simulink model "QPSK_Tx_HDL"  (R2017b)
settings: Solver=FixedStepDiscrete  StartTime=0.0  StopTime=inf  RelTol=1e-3
PreLoadFcn:
  | sdrzQPSKTxFPGA_params = QPSK_Tx_HDL_init;
InitFcn:
  | sdrzQPSKTxFPGA_params = QPSK_Tx_HDL_init;
libraries: hdlsllib x3, dspsigops x2, adirfsom_lib x1, commrandsrc3 x1, commsequence2 x1, dspmlti4 x1, commdigbbndpm3 x1
CloseFcn:
  | clear sdrzQPSKTxFPGA_params;
Description:
  | This model is used to generate a targeted .bit for an SDR platform
settings Model: DataTypeOverride=Off  ModifiedByFormat=The MathWorks Inc.  SimulationMode=accelerator  Creator=The MathWorks, Inc.  LastModifiedBy=The MathWorks Inc.
settings DataIOCC: LimitDataPoints=on  SaveFormat=Array  SaveOutput=off  SaveTime=off
settings OptimizationCC: BlockReduction=off  ConditionallyExecuteInputs=off  DefaultParameterBehavior=Inlined  LifeSpan=inf
settings DebuggingCC: AlgebraicLoopMsg=error  UnderspecifiedInitializationDetection=Classic  MergeDetectMultiDrivingBlocksExec=none  SolverPrmCheckMsg=warning  MultiTaskDSMMsg=warning  MultiTaskCondExecSysMsg=none  SingleTaskRateTransMsg=error  ParameterPrecisionLossMsg=none  AllowSymbolicDim=off  StateNameClashWarn=warning  SFUnexpectedBacktrackingDiag=warning  SFNoUnconditionalDefaultTransitionDiag=warning  SFExecutionAtInitializationDiag=none
settings HardwareCC: ProdBitPerPointer=32  ProdBitPerSizeT=32  ProdBitPerPtrDiffT=32  ProdLargestAtomicFloat=None  ProdIntDivRoundTo=Undefined  ProdEndianess=Unspecified  ProdWordSize=32  ProdHWDeviceType=ASIC/FPGA->ASIC/FPGA  TargetBitPerPointer=64  TargetBitPerSizeT=64  TargetBitPerPtrDiffT=64  TargetLongLongMode=on  TargetIntDivRoundTo=Zero  TargetEndianess=LittleEndian  TargetWordSize=64  TargetHWDeviceType=Generic->MATLAB Host Computer  ProdEqTarget=off
settings ModelReferenceCC: PropagateSignalLabelsOutOfModel=off
settings CodeAppCC: StateflowObjectComments=on
settings GRTTargetCC: TargetLangStandard=C89/C90 (ANSI)  GeneratePreprocessorConditionals=Disable all
settings ConfigComp: CovMetricSettings=dw  CovHtmlReporting=on  CovSaveCumulativeToWorkspaceVar=on  CovSaveSingleToWorkspaceVar=on  CovExternalEMLEnable=off  CovSFcnEnable=off

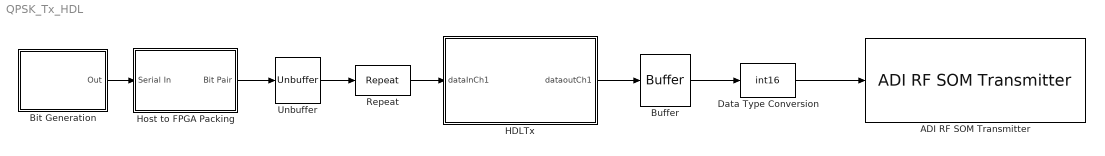
== system QPSK_Tx_HDL ==
  ADI RF SOM Transmitter : adirfsom_lib/ADI RF SOM Transmitter  IPAddress=192.168.3.2  CenterFrequencySource=Dialog  CenterFrequency=2400000000  GainSource=Dialog  Gain=-10  ChannelMapping=1  BasebandSampleRate=sdrzQPSKTxFPGA_params.RadioFrontEndSampleRate  EnableBurstMode=off  NumFramesInBurst=20  DMATimeoutValue=1  EnableTxPrimingMode=on  blockMode=Normal  LostSamplesOutputPort=off  OverflowOutputPort=off  SimulateUsing=Code generation  DataSourceSelect=Host  DDSFrequency=[ 1000000, 1000000; 1000000, 1000000 ]  DDSPhase=[ 0, 0; 0, 0 ]  DDSScale=[ 250000, 250000; 250000, 250000 ]  BypassUserLogic=on  ShowAdvancedProperties=on  ShowInternalProperties=off  subDeviceList=zynqTransmitter  sdrExecutionMode=HW  dataUDPPort=-1  ctrlUDPPort=-1  FIRCoefficientSize=[ 128; 128 ]  FIRCoefficients=[ 55, -54, 42, -126, -123, -317, -399, -581, -646, -711, -634, -507, -263, -10, 255, 424, 492, 401, 201, -84, -352, -540, -566, -423, -126, 234, 562, 738, 701, 429, -5, -490, -866, -1007, -834, -372, 266, 891, 1301, 1334, 936, 178, -733, -1524, -1917, -1731, -944, 274, 1590, 2585, 2881, 2255, 741, -1344, -3435, -4850, -4942, -3285, 197, 5169, 10923, 16509, 20932, 23375, 23375, 20932, 16509, 10923, 5169, 197, -3285, -4942, -4850, -3435, -1344, 741, 2255, 2881, 2585, 1590, 274, -944, -1731, -1917, -1524, -733, 178, 936, 1334, 1301, 891, 266, -372, -834, -1007, -866, -490, -5, 429, 701, 738, 562, 234, -126, -423, -566, -540, -352, -84, 201, 401, 492, 424, 255, -10, -263, -507, -634, -711, -646, -581, -399, -317, -123, -126, 42, -54, 55; 190, -88, 329, -40, 239, -99, -24, -349, -377, -611, -573, -604, -395, -229, 66, 239, 394, 350, 227, -46, -300, -534, -593, -506, -221, 137, 512, 737, 765, 526, 103, -420, -852, -1069, -947, -512, 156, 841, 1341, 1450, 1100, 333, -638, -1531, -2028, -1922, -1152, 115, 1544, 2677, 3099, 2535, 997, -1205, -3479, -5095, -5345, -3750, -199, 4965, 11002, 16895, 21580, 24172, 24172, 21580, 16895, 11002, 4965, -199, -3750, -5345, -5095, -3479, -1205, 997, 2535, 3099, 2677, 1544, 115, -1152, -1922, -2028, -1531, -638, 333, 1100, 1450, 1341, 841, 156, -512, -947, -1069, -852, -420, 103, 526, 765, 737, 512, 137, -221, -506, -593, -534, -300, -46, 227, 350, 394, 239, 66, -229, -395, -604, -573, -611, -377, -349, -24, -99, 239, -40, 329, -88, 190 ]  FIRGain=[ 0; -12 ]  FIRDecimInterpFactor=[ 4; 4 ]  AnalogFilterCutoff=[ 3152524; 3161715 ]  FilterPathRates=[ 983040000, 122880000, 61440000, 30720000, 15360000, 3840000; 983040000, 122880000, 61440000, 30720000, 15360000, 3840000 ]  FilterDesignTypeForTx=DefaultFilter  FilterDesignTypeForRx=DefaultFilterFromOther
      settings: SourceProductName=Communications System Toolbox Support Package for Xilinx Zynq-Based Radio
  Bit Generation : Subsystem
      mask Display: disp('Bits Generation')
  Buffer : Buffer  N=4000  OutputFrames=off
  Data Type Conversion : DataTypeConversion  OutDataTypeStr=int16  ConvertRealWorld=Stored Integer (SI)
  HDLTx : Subsystem
  Host to FPGA Packing : Subsystem
  Repeat : dspsigops/Repeat  N=sdrzQPSKTxFPGA_params.Upsampling  RateOptions=Allow multirate processing  ic=0  mode=Unused parameter value
      settings: SourceProductName=DSP System Toolbox
  Unbuffer : Unbuffer
  wires:
  Unbuffer/1 -> Repeat/1
  Bit Generation/1(Out) -> Host to FPGA Packing/1(Serial In)
  Buffer/1 -> Data Type Conversion/1
  HDLTx/1(dataoutCh1) -> Buffer/1
  Host to FPGA Packing/1(Bit Pair) -> Unbuffer/1
  Repeat/1 -> HDLTx/1(dataInCh1)
  Data Type Conversion/1 -> ADI RF SOM Transmitter/1

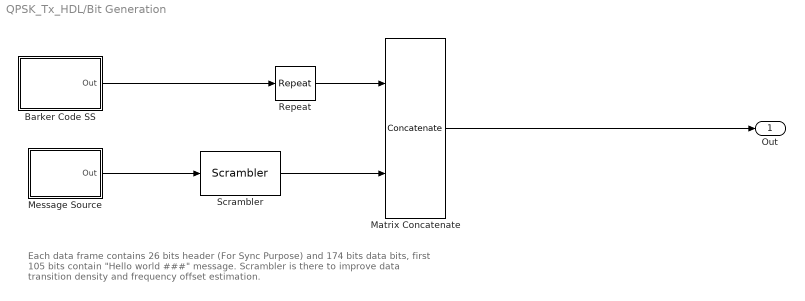
== system QPSK_Tx_HDL/Bit Generation ==
  note: Each data frame contains 26 bits header (For Sync Purpose) and 174 bits data bits,
      | first 105 bits contain "Hello world ###" message. Scrambler is there to improve data
      | transition density and frequency offset estimation.
  Barker Code SS : Subsystem
      mask Display: disp('Unipolar\nBarker Code')
  Matrix Concatenate : Concatenate  Mode=Multidimensional array
  Message Source : Subsystem
      mask Display: disp('Message\nSource')
  Repeat : dspsigops/Repeat  N=2  InputProcessing=Columns as channels (frame based)  RateOptions=Enforce single-rate processing  ic=0  mode=Unused parameter value
      settings: SourceProductName=DSP System Toolbox
  Scrambler : commsequence2/Scrambler  M=2  poly=[1 1 1 0 1]  iniStaSource=Dialog Parameter  ini_sta=[0 0 0 0]  resetViaPort=off
      settings: SourceProductName=Communications System Toolbox  SourceProductBaseCode=CM
  Out : Outport
  wires:
  Message Source/1(Out) -> Scrambler/1
  Scrambler/1 -> Matrix Concatenate/2
  Repeat/1 -> Matrix Concatenate/1
  Barker Code SS/1(Out) -> Repeat/1
  Matrix Concatenate/1 -> Out/1

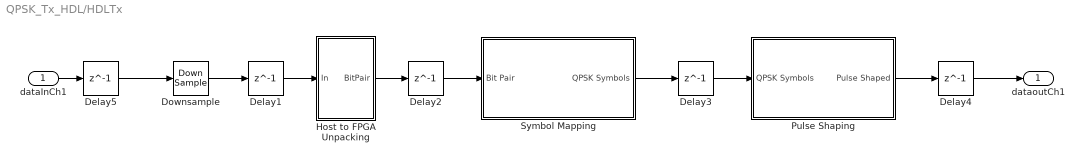
== system QPSK_Tx_HDL/HDLTx ==
  dataInCh1 : Inport
  Delay{1..5} (5 alike) : Delay  DelayLength=1  InitialCondition=0
  Downsample : DownSample  N=sdrzQPSKTxFPGA_params.Upsampling  RateOptions=Allow multirate processing
  Host to FPGA Unpacking : Subsystem
  Pulse Shaping : Subsystem
  Symbol Mapping : Subsystem
  dataoutCh1 : Outport
  wires:
  Delay3/1 -> Pulse Shaping/1(QPSK Symbols)
  Pulse Shaping/1(Pulse Shaped) -> Delay4/1
  Delay4/1 -> dataoutCh1/1
  Delay1/1 -> Host to FPGA Unpacking/1(In)
  dataInCh1/1 -> Delay5/1
  Delay2/1 -> Symbol Mapping/1(Bit Pair)
  Host to FPGA Unpacking/1(BitPair) -> Delay2/1
  Symbol Mapping/1(QPSK Symbols) -> Delay3/1
  Delay5/1 -> Downsample/1
  Downsample/1 -> Delay1/1

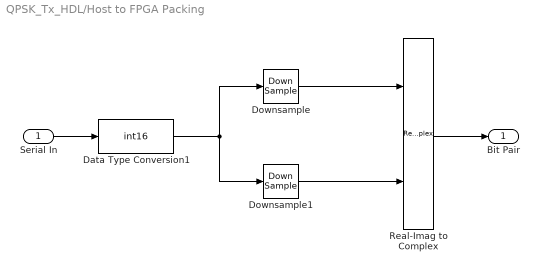
== system QPSK_Tx_HDL/Host to FPGA Packing ==
  Serial In : Inport
  Data Type Conversion1 : DataTypeConversion  OutDataTypeStr=int16
  Downsample : DownSample  RateOptions=Allow multirate processing
  Downsample1 : DownSample  phase=1  RateOptions=Allow multirate processing
  Real-Imag to Complex : RealImagToComplex
  Bit Pair : Outport
  wires:
  Downsample/1 -> Real-Imag to Complex/1
  Serial In/1 -> Data Type Conversion1/1
  Data Type Conversion1/1 -> Downsample1/1, Downsample/1
  Downsample1/1 -> Real-Imag to Complex/2
  Real-Imag to Complex/1 -> Bit Pair/1

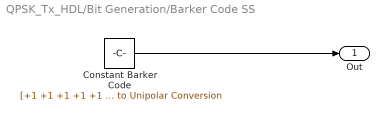
== system QPSK_Tx_HDL/Bit Generation/Barker Code SS ==
  Constant Barker Code : Constant  Value=|  VectorParams1D=off  OutDataTypeStr=double
      | [+1 +1 +1 +1 +1 -1 -1 +1 +1 -1 +1 -1 +1
      | ].' > 0  % Bipolar to Unipolar Conversion
  Out : Outport
  wires:
  Constant Barker Code/1 -> Out/1

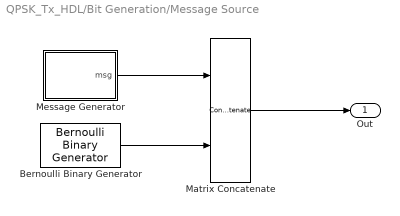
== system QPSK_Tx_HDL/Bit Generation/Message Source ==
  Bernoulli Binary Generator : commrandsrc3/Bernoulli Binary Generator  ProbabilityOfZero=0.5  SeedSource=Parameter  Seed=61  SampleTime=sdrzQPSKTxFPGA_params.FrameTime / (sdrzQPSKTxFPGA_params.DataLength - sdrzQPSKTxFPGA_params.MsgLength)  SamplesPerFrame=sdrzQPSKTxFPGA_params.DataLength - sdrzQPSKTxFPGA_params.MsgLength  OutputDataType=double  SimulateUsing=Interpreted execution
  Matrix Concatenate : Concatenate  Mode=Multidimensional array
  Message Generator : MATLAB Function  TreatAsAtomicUnit=on
  Out : Outport
  wires:
  Matrix Concatenate/1 -> Out/1
  Bernoulli Binary Generator/1 -> Matrix Concatenate/2
  Message Generator/1(msg) -> Matrix Concatenate/1

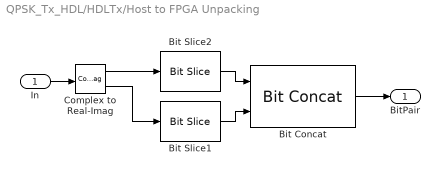
== system QPSK_Tx_HDL/HDLTx/Host to FPGA Unpacking ==
  In : Inport
  Bit Concat : hdlsllib/Logic and Bit Operations/Bit Concat  numInputs=2
      settings: SourceProductName=HDL Coder  SourceProductBaseCode=HD
  Bit Slice1 : hdlsllib/Logic and Bit Operations/Bit Slice  lidx=0  ridx=0
  Bit Slice2 : hdlsllib/Logic and Bit Operations/Bit Slice  lidx=0  ridx=0
  Complex to Real-Imag : ComplexToRealImag
  BitPair : Outport
  wires:
  Complex to Real-Imag/1 -> Bit Slice2/1
  In/1 -> Complex to Real-Imag/1
  Complex to Real-Imag/2 -> Bit Slice1/1
  Bit Slice2/1 -> Bit Concat/1
  Bit Slice1/1 -> Bit Concat/2
  Bit Concat/1 -> BitPair/1

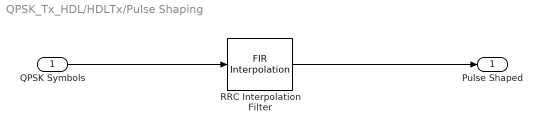
== system QPSK_Tx_HDL/HDLTx/Pulse Shaping ==
  QPSK Symbols : Inport
  RRC Interpolation Filter : dspmlti4/FIR Interpolation  FilterSource=Dialog parameters  h=sdrzQPSKTxFPGA_params.TransmitterFilterCoefficients  L=sdrzQPSKTxFPGA_params.Upsampling  FilterObject=Htxrc  framing=Allow multirate processing  outputBufInitCond=0  roundingMode=Floor  overflowMode=off  firstCoeffMode=Specify word length  firstCoeffWordLength=16  firstCoeffFracLength=15  firstCoeffDataTypeStr=fixdt(1,16)  firstCoeffMin=[]  firstCoeffMax=[]  firstCoeffLastDataTypeStr=fixdt(1,16)  prodOutputMode=Binary point scaling  prodOutputWordLength=31  prodOutputFracLength=29  prodOutputDataTypeStr=fixdt(1,31,29)  prodOutputLastDataTypeStr=fixdt(1,31,29)  accumMode=Binary point scaling  accumWordLength=33  accumFracLength=29  accumDataTypeStr=fixdt(1,33,29)  accumLastDataTypeStr=fixdt(1,33,29)  outputMode=Binary point scaling  outputWordLength=16  outputFracLength=14  outputDataTypeStr=fixdt(1,16,14)  outputMin=[]  outputMax=[]  outputLastDataTypeStr=fixdt(1,16,14)
      settings: SourceProductName=DSP System Toolbox
  Pulse Shaped : Outport
  wires:
  QPSK Symbols/1 -> RRC Interpolation Filter/1
  RRC Interpolation Filter/1 -> Pulse Shaped/1

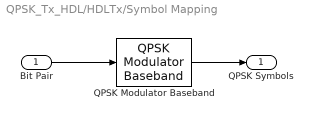
== system QPSK_Tx_HDL/HDLTx/Symbol Mapping ==
  Bit Pair : Inport
  QPSK Modulator Baseband : commdigbbndpm3/QPSK Modulator Baseband  InType=Integer  Enc=Gray  Ph=pi/4  outDtype=Fixed-point  outWordLen=16  outUDDataType=sfix(16)  outFracLenMode=User-defined  outFracLen=15  outDataTypeStr=fixdt(1,16,15)  outLastDataTypeStr=fixdt(1,16,15)
  QPSK Symbols : Outport
  wires:
  QPSK Modulator Baseband/1 -> QPSK Symbols/1
  Bit Pair/1 -> QPSK Modulator Baseband/1

== matlab function QPSK_Tx_HDL/Bit Generation/Message Source/Message Generator ==
  data: msg output size=[sdrzQPSKTxFPGA_params.MsgLength,1]
function msg = genMsg
%#codegen
persistent msgStrSet count;
if isempty(msgStrSet)
    count = 0;
    msgStrSet = ['Hello world 000';...
              'Hello world 001';...
              'Hello world 002';...
              'Hello world 003';...
              'Hello world 004';...
              'Hello world 005';...
              'Hello world 006';...
              'Hello world 007';...
              'Hello world 008';...
              'Hello world 009';...
              'Hello world 010';...
              'Hello world 011';...
              'Hello world 012';...
              'Hello world 013';...
              'Hello world 014';...
              'Hello world 015';...
              'Hello world 016';...
              'Hello world 017';...
              'Hello world 018';...
              'Hello world 019';...
              'Hello world 020';...
              'Hello world 021';...
              'Hello world 022';...
              'Hello world 023';...
              'Hello world 024';...
              'Hello world 025';...
              'Hello world 026';...
              'Hello world 027';...
              'Hello world 028';...
              'Hello world 029';...
              'Hello world 030';...
              'Hello world 031';...
              'Hello world 032';...
              'Hello world 033';...
              'Hello world 034';...
              'Hello world 035';...
              'Hello world 036';...
              'Hello world 037';...
              'Hello world 038';...
              'Hello world 039';...
              'Hello world 040';...
              'Hello world 041';...
              'Hello world 042';...
              'Hello world 043';...
              'Hello world 044';...
              'Hello world 045';...
              'Hello world 046';...
              'Hello world 047';...
              'Hello world 048';...
              'Hello world 049';...
              'Hello world 050';...
              'Hello world 051';...
              'Hello world 052';...
              'Hello world 053';...
              'Hello world 054';...
              'Hello world 055';...
              'Hello world 056';...
              'Hello world 057';...
              'Hello world 058';...
              'Hello world 059';...
              'Hello world 060';...
              'Hello world 061';...
              'Hello world 062';...
              'Hello world 063';...
              'Hello world 064';...
              'Hello world 065';...
              'Hello world 066';...
              'Hello world 067';...
              'Hello world 068';...
              'Hello world 069';...
              'Hello world 070';...
              'Hello world 071';...
              'Hello world 072';...
              'Hello world 073';...
              'Hello world 074';...
              'Hello world 075';...
              'Hello world 076';...
              'Hello world 077';...
              'Hello world 078';...
              'Hello world 079';...
              'Hello world 080';...
              'Hello world 081';...
              'Hello world 082';...
              'Hello world 083';...
              'Hello world 084';...
              'Hello world 085';...
              'Hello world 086';...
              'Hello world 087';...
              'Hello world 088';...
              'Hello world 089';...
              'Hello world 090';...
              'Hello world 091';...
              'Hello world 092';...
              'Hello world 093';...
              'Hello world 094';...
              'Hello world 095';...
              'Hello world 096';...
              'Hello world 097';...
              'Hello world 098';...
              'Hello world 099'];              
end
msgStr = msgStrSet(count+1,:);
msgBin = de2bi(int8(msgStr),7,'left-msb');
msg = reshape(double(msgBin).',105,1);
count = mod(count+1,100);
